simulink library "MFMdl3"  (Simulink 8.8)
settings: Solver=VariableStepAuto  StartTime=0.0  StopTime=10.0  RelTol=1e-3
libraries: simulink x2
settings Model: Creator=viett  LastModifiedBy=viett

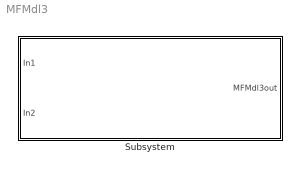
== system MFMdl3 ==
  Subsystem : Subsystem

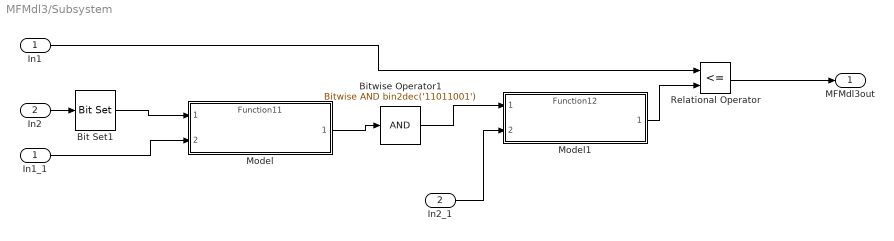
== system MFMdl3/Subsystem ==
  In1 : Inport
  In2 : Inport  Port=2
  Bit Set1 : simulink/Logic and Bit Operations/Bit Set  iBit=0
  Bitwise Operator1 : simulink/Logic and Bit Operations/Bitwise Operator  logicop=AND  UseBitMask=on  BitMask=bin2dec('11011001')  BitMaskRealWorld=Stored Integer
  In1_1 : InportShadow
  In2_1 : InportShadow  Port=2
  Model : ModelReference  ModelNameDialog=Function11.slx  SimulationMode=Normal  ModelReferenceVersion=1.20
  Model1 : ModelReference  ModelNameDialog=Function12.slx  SimulationMode=Normal  ModelReferenceVersion=1.18
  Relational Operator : RelationalOperator  Operator=<=  OutDataTypeStr=boolean  RndMeth=Simplest
  MFMdl3out : Outport
  wires:
  Model/1 -> Bitwise Operator1/1
  Bit Set1/1 -> Model/1
  In1/1 -> Relational Operator/1
  In1_1/1 -> Model/2
  Model1/1 -> Relational Operator/2
  In2/1 -> Bit Set1/1
  Relational Operator/1 -> MFMdl3out/1
  Bitwise Operator1/1 -> Model1/1
  In2_1/1 -> Model1/2
